simulink model "main_observer_sim2"  (R2015a)
settings: Solver=ode45  StartTime=0.0  StopTime=10  FixedStep=1e-4  MaxStep=1e-3  RelTol=1e-3
values from neighbouring files (symbols this model uses):
  A = sys_rand.A    [main_Observer_states.m]
  B = B(:,1:end-1)    [main_Observer_states.m]
  beta = [5657.83678507 -1913.14902282 -932.285352789 348.153105943 2507.13858904 -2140.9545479]    [beta.mat]    (also in main_disturbance_observer.m = inv(delta2)*beta_hat)
  C = [0.617255113405149,0,0,-0.448535555941661,0.134230346538703,1.41932930409004;0.283640603624291,0,2.22808153625508,-1.86462753317668,-1.99763494036701,-0.0116516666362024;0.350975702033898,-0.174162030842294,1.44167650824058,-0.392420914284623,1.30288133017051,-0.392171726620127]    [finding_Y.m]    (also in main_Observer_states.m = sys_rand.C)
  Delta = (eye(n,n)+(-H*CHp+Y*(eye(p,p)-(C*H)*CHp))*C)*B    [main_Observer_states.m]    (also in observer.mat = [-0.0673817558455 0.158220969334 -1.63112233705 -0.121104966)
  Gama = eta*A-X*C    [main_Observer_states.m]    (also in observer.mat = [-0.665415381788 -1.71297839543 -11.0757301234 9.21615917151)
  H = B(:,end)    [main_Observer_states.m]
  Phi = dec2mat(LMISYS,xopt,2)    [main_Observer_states.m]    (also in observer.mat = [2.03974430811 -0.144807404976 -3.64797116197 7.53997403465 )
  theta = theta1+Y*theta2    [main_Observer_states.m]    (also in observer.mat = [-0.848682280391 0.936204937086 2.9983152382 2.21151006385 4)
settings Model: Creator=p4wp4w  LastModifiedBy=p4wp4w

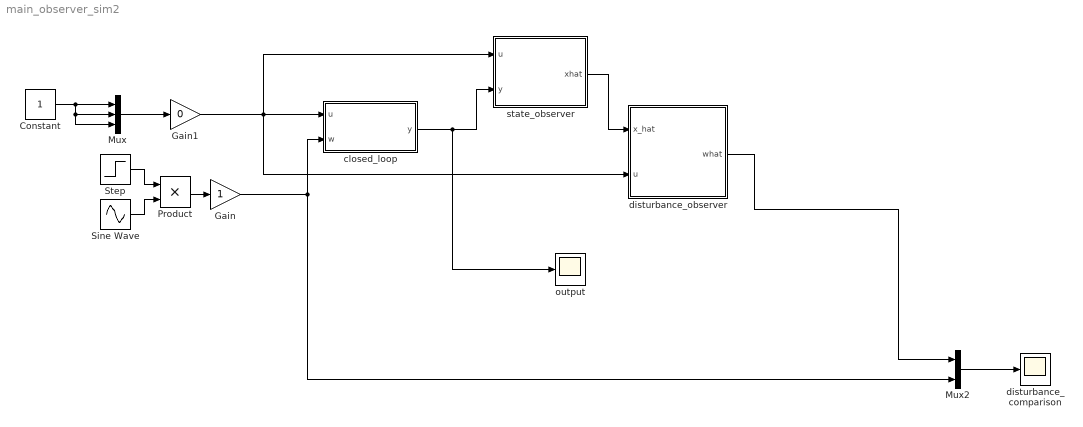
== system main_observer_sim2 ==
  Constant : Constant
  Gain : Gain
  Gain1 : Gain  Gain=0
  Mux : Mux  Inputs=3
  Mux2 : Mux  Inputs=2
  Product : Product
  Sine Wave : Sin  Frequency=10  SampleTime=0
  Step : Step  Before=8  After=0  SampleTime=0
  closed_loop : Subsystem
  disturbance_comparison : Scope
      settings: ShowLegends=on  YMin=-50  YMax=850
  disturbance_observer : Subsystem
  output : Scope
      settings: YMin=-0.0024  YMax=-2.1684e-19  SaveName=ScopeData5
  state_observer : Subsystem
  wires:
  Gain1/1 -> disturbance_observer/2(u), state_observer/1(u), closed_loop/1(u)
  closed_loop/1(y) -> output/1, state_observer/2(y)
  Mux2/1 -> disturbance_comparison/1
  disturbance_observer/1(what) -> Mux2/1
  Gain/1 -> Mux2/2, closed_loop/2(w)
  state_observer/1(xhat) -> disturbance_observer/1(x_hat)
  Product/1 -> Gain/1
  Step/1 -> Product/1
  Sine Wave/1 -> Product/2
  Mux/1 -> Gain1/1
  Constant/1 -> Mux/2, Mux/3, Mux/1

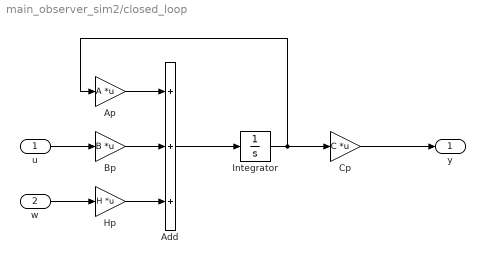
== system main_observer_sim2/closed_loop ==
  u : Inport
  w : Inport  Port=2
  Add : Sum  Inputs=+++
  Ap : Gain  Gain=A  Multiplication=Matrix(K*u)
  Bp : Gain  Gain=B  Multiplication=Matrix(K*u)
  Cp : Gain  Gain=C  Multiplication=Matrix(K*u)
  Hp : Gain  Gain=H  Multiplication=Matrix(K*u)
  Integrator : Integrator
  y : Outport
  wires:
  w/1 -> Hp/1
  u/1 -> Bp/1
  Add/1 -> Integrator/1
  Bp/1 -> Add/2
  Integrator/1 -> Cp/1, Ap/1
  Ap/1 -> Add/1
  Hp/1 -> Add/3
  Cp/1 -> y/1

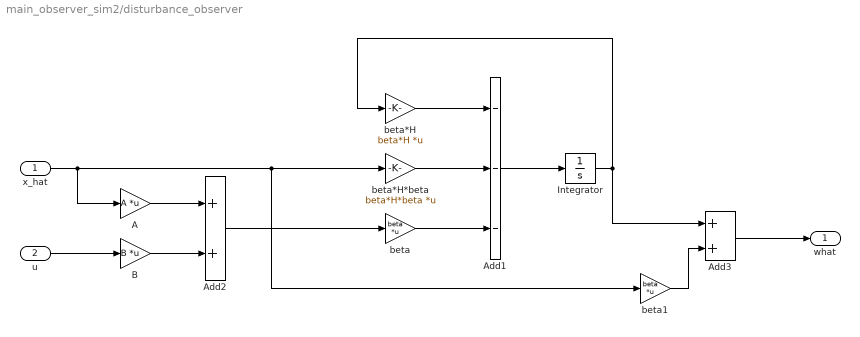
== system main_observer_sim2/disturbance_observer ==
  x_hat : Inport
  u : Inport  Port=2
  A : Gain  Gain=A  Multiplication=Matrix(K*u)
  Add1 : Sum  Inputs=---
  Add2 : Sum
  Add3 : Sum
  B : Gain  Gain=B  Multiplication=Matrix(K*u)
  Integrator : Integrator
  beta : Gain  Gain=beta  Multiplication=Matrix(K*u)
  beta*H : Gain  Gain=beta*H  Multiplication=Matrix(K*u)
  beta*H*beta : Gain  Gain=beta*H*beta  Multiplication=Matrix(K*u)
  beta1 : Gain  Gain=beta  Multiplication=Matrix(K*u)
  what : Outport
  wires:
  Add1/1 -> Integrator/1
  beta*H/1 -> Add1/1
  Integrator/1 -> Add3/1, beta*H/1
  beta*H*beta/1 -> Add1/2
  x_hat/1 -> A/1, beta1/1, beta*H*beta/1
  beta/1 -> Add1/3
  A/1 -> Add2/1
  B/1 -> Add2/2
  u/1 -> B/1
  Add2/1 -> beta/1
  beta1/1 -> Add3/2
  Add3/1 -> what/1

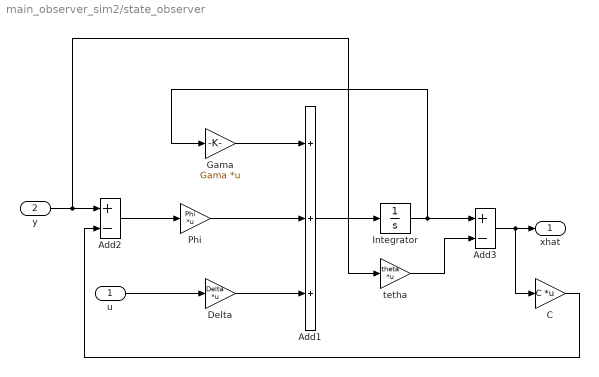
== system main_observer_sim2/state_observer ==
  u : Inport
  y : Inport  Port=2
  Add1 : Sum  Inputs=+++
  Add2 : Sum  Inputs=+-
  Add3 : Sum  Inputs=+-
  C : Gain  Gain=C  Multiplication=Matrix(K*u)
  Delta : Gain  Gain=Delta  Multiplication=Matrix(K*u)
  Gama : Gain  Gain=Gama  Multiplication=Matrix(K*u)
  Integrator : Integrator
  Phi : Gain  Gain=Phi  Multiplication=Matrix(K*u)
  tetha : Gain  Gain=theta  Multiplication=Matrix(K*u)
  xhat : Outport
  wires:
  y/1 -> tetha/1, Add2/1
  C/1 -> Add2/2
  Add1/1 -> Integrator/1
  Gama/1 -> Add1/1
  Integrator/1 -> Gama/1, Add3/1
  Phi/1 -> Add1/2
  Add2/1 -> Phi/1
  u/1 -> Delta/1
  Delta/1 -> Add1/3
  tetha/1 -> Add3/2
  Add3/1 -> C/1, xhat/1
